simulink model "Bias_TestGen9"  (R2017b)
settings: Solver=FixedStepDiscrete  StartTime=0.0  StopTime=10.0  RelTol=1e-3
undefined symbols (not defined in the file): Block_TestLib, enable
settings Model: Creator=hbourbou  LastModifiedBy=hbourbou
settings DebuggingCC: ParameterOverflowMsg=none

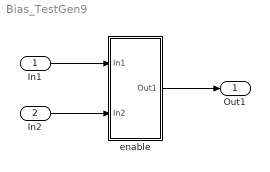
== system Bias_TestGen9 ==
  In1 : Inport
  In2 : Inport  Port=2
  enable : Subsystem  AncestorBlock=Block_TestLib/enable
  Out1 : Outport
  wires:
  In1/1 -> enable/1(In1)
  In2/1 -> enable/2(In2)
  enable/1(Out1) -> Out1/1

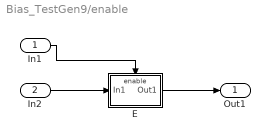
== system Bias_TestGen9/enable ==
  In1 : Inport  OutDataTypeStr=boolean
  In2 : Inport  Port=2
  E : Subsystem  TreatAsAtomicUnit=on
  Out1 : Outport
  wires:
  In1/1 -> E/Enable
  In2/1 -> E/1(In1)
  E/1(Out1) -> Out1/1

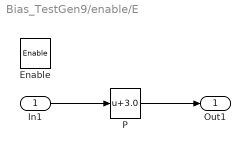
== system Bias_TestGen9/enable/E ==
  In1 : Inport  OutDataTypeStr=uint8  PortDimensions=[1 3]
  Enable : EnablePort
  P : Bias  Bias=3.0
  Out1 : Outport
  wires:
  In1/1 -> P/1
  P/1 -> Out1/1
